simulink model "rovSim_los"  (R2017a)
settings: Solver=ode4  StartTime=0.0  StopTime=10.0  FixedStep=mdl.tStep  RelTol=1e-3
undefined symbols (not defined in the file): ics, kdd, kds, kdu, kid, kis, kiu, kpd, kps, kpu, magnitude, n_max, r, rov, Tinv, ud, v_c, waypoints
libraries: simulink x4
settings Model: Creator=e_anderlini  LastModifiedBy=e_anderlini

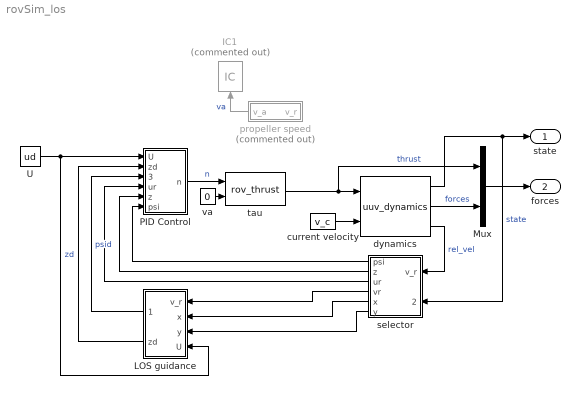
== system rovSim_los ==
  IC1 : InitialCondition  Commented=on  Value=0
  LOS guidance : Subsystem
  Mux : Mux  Inputs=[6,18]
  PID Control : Subsystem
  U : Constant  Value=ud
  current velocity : Constant  Value=v_c
  dynamics : S-Function  FunctionName=uuv_dynamics  Parameters=rov.weight,rov.buoyancy,rov.G,rov.B,ics,rov.inv_mass',rov.M_A',rov.M_RB',rov.D_L',rov.D_q'  SFunctionDeploymentMode=off  EnableBusSupport=off
  propeller speed : Subsystem  Commented=on
  selector : Subsystem
  tau : S-Function  FunctionName=rov_thrust  Parameters=rov.density,rov.prop_diam,rov.K_T,rov.theta,rov.T'  SFunctionDeploymentMode=off  EnableBusSupport=off
  va : Constant  Value=0
  state : Outport
  forces : Outport  Port=2
  wires:
  dynamics/1 -> selector/2(states), state/1  "state"
  tau/1 -> Mux/1, dynamics/1  "thrust"
  Mux/1 -> forces/1
  dynamics/2 -> Mux/2  "forces"
  propeller speed/1(v_a) -> IC1/1  "va"
  PID Control/1(n) -> tau/1  "n"
  va/1 -> tau/2
  selector/3(ur) -> PID Control/4(ur)
  dynamics/3 -> selector/1(v_r)  "rel_vel"
  selector/2(z) -> PID Control/5(z)
  selector/1(psi) -> PID Control/6(psi)
  current velocity/1 -> dynamics/2
  U/1 -> LOS guidance/4(U), PID Control/1(U)
  selector/4(vr) -> LOS guidance/1(v_r)
  selector/5(x) -> LOS guidance/2(x)
  selector/6(y) -> LOS guidance/3(y)
  LOS guidance/2(zd) -> PID Control/2(zd)  "zd"
  LOS guidance/1(psid) -> PID Control/3(psid)  "psid"

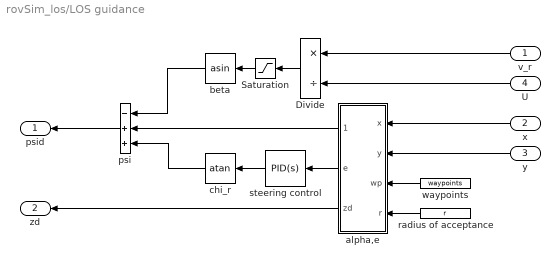
== system rovSim_los/LOS guidance ==
  v_r : Inport
  x : Inport  Port=2
  y : Inport  Port=3
  U : Inport  Port=4
  Divide : Product  Inputs=*/
  Saturation : Saturate  UpperLimit=1  LowerLimit=-1
  alpha,e : MATLAB Function  TreatAsAtomicUnit=on
  beta : Trigonometry  Operator=asin
  chi_r : Trigonometry  Operator=atan
  psi : Sum  Inputs=-++
  radius of acceptance : Constant  Value=r
  steering control : simulink/Continuous/PID Controller  Controller=PID  TimeDomain=Continuous-time  SampleTime=-1  IntegratorMethod=Forward Euler  FilterMethod=Forward Euler  Form=Parallel  UseFilter=on  ControllerParametersSource=internal  P=kps  I=kis  D=kds  N=100  InitialConditionSource=internal  InitialConditionForIntegrator=0  InitialConditionForFilter=0  ExternalReset=none  LimitOutput=off  UpperSaturationLimit=inf  LowerSaturationLimit=-inf  LinearizeAsGain=on  AntiWindupMode=none  Kb=1  TrackingMode=off  Kt=1  PParamMin=[]  PParamMax=[]  IParamMin=[]  IParamMax=[]  DParamMin=[]  DParamMax=[]  NParamMin=[]  NParamMax=[]  KbParamMin=[]  KbParamMax=[]  KtParamMin=[]  KtParamMax=[]  POutMin=[]  POutMax=[]  IOutMin=[]  IOutMax=[]  DOutMin=[]  DOutMax=[]  NOutMin=[]  NOutMax=[]  KbOutMin=[]  KbOutMax=[]  KtOutMin=[]  KtOutMax=[]  IntegratorOutMin=[]  IntegratorOutMax=[]  FilterOutMin=[]  FilterOutMax=[]  SumOutMin=[]  SumOutMax=[]  SumI1OutMin=[]  SumI1OutMax=[]  SumI2OutMin=[]  SumI2OutMax=[]  SumI3OutMin=[]  SumI3OutMax=[]  SumDOutMin=[]  SumDOutMax=[]  SaturationOutMin=[]  SaturationOutMax=[]  IntegratorContinuousStateAttributes=''  IntegratorStateMustResolveToSignalObject=off  IntegratorRTWStateStorageClass=Auto  FilterContinuousStateAttributes=''  FilterStateMustResolveToSignalObject=off  FilterRTWStateStorageClass=Auto  DifferentiatorICPrevScaledInput=0  DifferentiatorOutMin=[]  DifferentiatorOutMax=[]  InitialConditionSetting=State (most efficient)
  waypoints : Constant  Value=waypoints
  psid : Outport
  zd : Outport  Port=2
  wires:
  x/1 -> alpha,e/1(x)
  waypoints/1 -> alpha,e/3(wp)
  alpha,e/3(zd) -> zd/1
  alpha,e/2(e) -> steering control/1
  U/1 -> Divide/2
  radius of acceptance/1 -> alpha,e/4(r)
  y/1 -> alpha,e/2(y)
  beta/1 -> psi/1
  v_r/1 -> Divide/1
  Divide/1 -> Saturation/1
  steering control/1 -> chi_r/1
  alpha,e/1(alpha) -> psi/2
  chi_r/1 -> psi/3
  psi/1 -> psid/1
  Saturation/1 -> beta/1

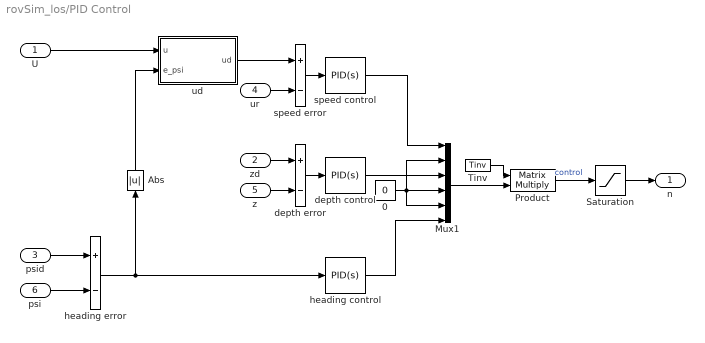
== system rovSim_los/PID Control ==
  U : Inport
  zd : Inport  Port=2
  psid : Inport  Port=3
  ur : Inport  Port=4
  z : Inport  Port=5
  psi : Inport  Port=6
  0 : Constant  Value=0
  Abs : Abs
  Mux1 : Mux  Inputs=6
  Product : Product  Multiplication=Matrix(*)
  Saturation : Saturate  UpperLimit=n_max  LowerLimit=-n_max
  Tinv : Constant  Value=Tinv  VectorParams1D=off
  depth control : simulink/Continuous/PID Controller  Controller=PID  TimeDomain=Continuous-time  SampleTime=-1  IntegratorMethod=Forward Euler  FilterMethod=Forward Euler  Form=Parallel  UseFilter=on  ControllerParametersSource=internal  P=kpd  I=kid  D=kdd  N=100  InitialConditionSource=internal  InitialConditionForIntegrator=0  InitialConditionForFilter=0  ExternalReset=none  LimitOutput=off  UpperSaturationLimit=inf  LowerSaturationLimit=-inf  LinearizeAsGain=on  AntiWindupMode=none  Kb=1  TrackingMode=off  Kt=1  PParamMin=[]  PParamMax=[]  IParamMin=[]  IParamMax=[]  DParamMin=[]  DParamMax=[]  NParamMin=[]  NParamMax=[]  KbParamMin=[]  KbParamMax=[]  KtParamMin=[]  KtParamMax=[]  POutMin=[]  POutMax=[]  IOutMin=[]  IOutMax=[]  DOutMin=[]  DOutMax=[]  NOutMin=[]  NOutMax=[]  KbOutMin=[]  KbOutMax=[]  KtOutMin=[]  KtOutMax=[]  IntegratorOutMin=[]  IntegratorOutMax=[]  FilterOutMin=[]  FilterOutMax=[]  SumOutMin=[]  SumOutMax=[]  SumI1OutMin=[]  SumI1OutMax=[]  SumI2OutMin=[]  SumI2OutMax=[]  SumI3OutMin=[]  SumI3OutMax=[]  SumDOutMin=[]  SumDOutMax=[]  SaturationOutMin=[]  SaturationOutMax=[]  IntegratorContinuousStateAttributes=''  IntegratorStateMustResolveToSignalObject=off  IntegratorRTWStateStorageClass=Auto  FilterContinuousStateAttributes=''  FilterStateMustResolveToSignalObject=off  FilterRTWStateStorageClass=Auto  DifferentiatorICPrevScaledInput=0  DifferentiatorOutMin=[]  DifferentiatorOutMax=[]  InitialConditionSetting=State (most efficient)
  depth error : Sum  Inputs=+-
  heading control : simulink/Continuous/PID Controller  Controller=PID  TimeDomain=Continuous-time  SampleTime=-1  IntegratorMethod=Forward Euler  FilterMethod=Forward Euler  Form=Parallel  UseFilter=on  ControllerParametersSource=internal  P=kpd  I=kid  D=kdd  N=100  InitialConditionSource=internal  InitialConditionForIntegrator=0  InitialConditionForFilter=0  ExternalReset=none  LimitOutput=off  UpperSaturationLimit=inf  LowerSaturationLimit=-inf  LinearizeAsGain=on  AntiWindupMode=none  Kb=1  TrackingMode=off  Kt=1  PParamMin=[]  PParamMax=[]  IParamMin=[]  IParamMax=[]  DParamMin=[]  DParamMax=[]  NParamMin=[]  NParamMax=[]  KbParamMin=[]  KbParamMax=[]  KtParamMin=[]  KtParamMax=[]  POutMin=[]  POutMax=[]  IOutMin=[]  IOutMax=[]  DOutMin=[]  DOutMax=[]  NOutMin=[]  NOutMax=[]  KbOutMin=[]  KbOutMax=[]  KtOutMin=[]  KtOutMax=[]  IntegratorOutMin=[]  IntegratorOutMax=[]  FilterOutMin=[]  FilterOutMax=[]  SumOutMin=[]  SumOutMax=[]  SumI1OutMin=[]  SumI1OutMax=[]  SumI2OutMin=[]  SumI2OutMax=[]  SumI3OutMin=[]  SumI3OutMax=[]  SumDOutMin=[]  SumDOutMax=[]  SaturationOutMin=[]  SaturationOutMax=[]  IntegratorContinuousStateAttributes=''  IntegratorStateMustResolveToSignalObject=off  IntegratorRTWStateStorageClass=Auto  FilterContinuousStateAttributes=''  FilterStateMustResolveToSignalObject=off  FilterRTWStateStorageClass=Auto  DifferentiatorICPrevScaledInput=0  DifferentiatorOutMin=[]  DifferentiatorOutMax=[]  InitialConditionSetting=State (most efficient)
  heading error : Sum  Inputs=+-
  speed control : simulink/Continuous/PID Controller  Controller=PID  TimeDomain=Continuous-time  SampleTime=-1  IntegratorMethod=Forward Euler  FilterMethod=Forward Euler  Form=Parallel  UseFilter=on  ControllerParametersSource=internal  P=kpu  I=kiu  D=kdu  N=100  InitialConditionSource=internal  InitialConditionForIntegrator=0  InitialConditionForFilter=0  ExternalReset=none  LimitOutput=off  UpperSaturationLimit=inf  LowerSaturationLimit=-inf  LinearizeAsGain=on  AntiWindupMode=none  Kb=1  TrackingMode=off  Kt=1  PParamMin=[]  PParamMax=[]  IParamMin=[]  IParamMax=[]  DParamMin=[]  DParamMax=[]  NParamMin=[]  NParamMax=[]  KbParamMin=[]  KbParamMax=[]  KtParamMin=[]  KtParamMax=[]  POutMin=[]  POutMax=[]  IOutMin=[]  IOutMax=[]  DOutMin=[]  DOutMax=[]  NOutMin=[]  NOutMax=[]  KbOutMin=[]  KbOutMax=[]  KtOutMin=[]  KtOutMax=[]  IntegratorOutMin=[]  IntegratorOutMax=[]  FilterOutMin=[]  FilterOutMax=[]  SumOutMin=[]  SumOutMax=[]  SumI1OutMin=[]  SumI1OutMax=[]  SumI2OutMin=[]  SumI2OutMax=[]  SumI3OutMin=[]  SumI3OutMax=[]  SumDOutMin=[]  SumDOutMax=[]  SaturationOutMin=[]  SaturationOutMax=[]  IntegratorContinuousStateAttributes=''  IntegratorStateMustResolveToSignalObject=off  IntegratorRTWStateStorageClass=Auto  FilterContinuousStateAttributes=''  FilterStateMustResolveToSignalObject=off  FilterRTWStateStorageClass=Auto  DifferentiatorICPrevScaledInput=0  DifferentiatorOutMin=[]  DifferentiatorOutMax=[]  InitialConditionSetting=State (most efficient)
  speed error : Sum  Inputs=+-
  ud : MATLAB Function  TreatAsAtomicUnit=on
  n : Outport
  wires:
  Product/1 -> Saturation/1  "control"
  0/1 -> Mux1/5, Mux1/2, Mux1/4
  Tinv/1 -> Product/1
  Saturation/1 -> n/1
  zd/1 -> depth error/1
  z/1 -> depth error/2
  depth error/1 -> depth control/1
  depth control/1 -> Mux1/3
  Mux1/1 -> Product/2
  speed error/1 -> speed control/1
  ur/1 -> speed error/2
  U/1 -> ud/1(u)
  speed control/1 -> Mux1/1
  psid/1 -> heading error/1
  psi/1 -> heading error/2
  heading error/1 -> Abs/1, heading control/1
  heading control/1 -> Mux1/6
  Abs/1 -> ud/2(e_psi)
  ud/1(ud) -> speed error/1

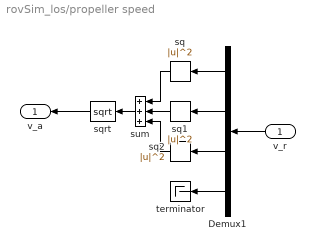
== system rovSim_los/propeller speed ==
  v_r : Inport
  Demux1 : Demux  Outputs=[1,1,1,3]
  sq : Math  Operator=magnitude^2  SaturateOnIntegerOverflow=on
  sq1 : Math  Operator=magnitude^2  SaturateOnIntegerOverflow=on
  sq2 : Math  Operator=magnitude^2  SaturateOnIntegerOverflow=on
  sqrt : Sqrt  SaturateOnIntegerOverflow=on
  sum : Sum  Inputs=+++
  terminator : Terminator
  v_a : Outport
  wires:
  sqrt/1 -> v_a/1
  Demux1/3 -> sq2/1
  Demux1/1 -> sq/1
  Demux1/2 -> sq1/1
  Demux1/4 -> terminator/1
  sq1/1 -> sum/2
  v_r/1 -> Demux1/1
  sum/1 -> sqrt/1
  sq/1 -> sum/1
  sq2/1 -> sum/3

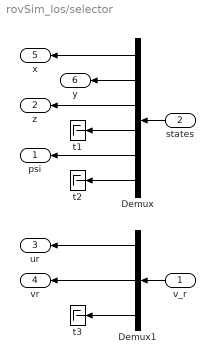
== system rovSim_los/selector ==
  v_r : Inport
  states : Inport  Port=2
  Demux : Demux  Outputs=[1,1,1,2,1,6]
  Demux1 : Demux  Outputs=[1,1,4]
  t1 : Terminator
  t2 : Terminator
  t3 : Terminator
  psi : Outport
  z : Outport  Port=2
  ur : Outport  Port=3
  vr : Outport  Port=4
  x : Outport  Port=5
  y : Outport  Port=6
  wires:
  Demux/4 -> t1/1
  Demux/1 -> x/1
  states/1 -> Demux/1
  Demux/3 -> z/1
  Demux/6 -> t2/1
  Demux/5 -> psi/1
  v_r/1 -> Demux1/1
  Demux1/1 -> ur/1
  Demux1/3 -> t3/1
  Demux/2 -> y/1
  Demux1/2 -> vr/1

== matlab function rovSim_los/LOS guidance/alpha,e ==
  data: x input; alpha output; y input; wp input; e output; r input; zd output
function [alpha,e,zd] = fcn(x,y,wp,r)
% fcn.m     e.anderlini@ucl.ac.uk      06/10/2017
%%%%%%%%%%%%%%%%%%%%%%%%%%%%%%%%%%%%%%%%%%%%%%%%%%%%%%%%%%%%%%%%%%%%%%%%%%%
% This function returns the angle alpha and the cross-track error.
% Input:
% x:  x-position;
% y:  y-position;
% wp: waypoints;
% r:  radius of acceptance.
%%%%%%%%%%%%%%%%%%%%%%%%%%%%%%%%%%%%%%%%%%%%%%%%%%%%%%%%%%%%%%%%%%%%%%%%%%%

persistent k n alp;
% Initialize persistent variables:
if isempty(k)
    k = 1;
    n = size(wp,1);
    alp = atan2(wp(2,2)-wp(1,2),wp(2,1)-wp(1,1));
end

% Check if k has to be updated:
if k<n-1
    if ((wp(k+1,1)-x)^2+(wp(k+1,2)-y)^2) <= r^2
        k = k + 1;
        alp = atan2(wp(k+1,2)-wp(k,2),wp(k+1,1)-wp(k,1));
    end
end

% Compute the cross-track error:
e = [-sin(alp),cos(alp)]*[wp(k,1)-x;wp(k,2)-y];
% Output the angle and desired depth as well:
alpha = alp;
zd = wp(k,3);

end

== matlab function rovSim_los/PID Control/ud ==
  data: u input; ud output; e_psi input
function ud = fcn(u,e_psi)

pi2 = pi/2;

if e_psi<pi2
    ud = u*(1-e_psi/pi2);
else
    ud = 0;
end

end
